simulink model "Dist_rej_lin"  (R2015b)
settings: Solver=VariableStepAuto  StartTime=0.0  StopTime=100  RelTol=1e-3
undefined symbols (not defined in the file): A, D
libraries: simulink x1
settings Model: Creator=Pramod  LastModifiedBy=Pramod

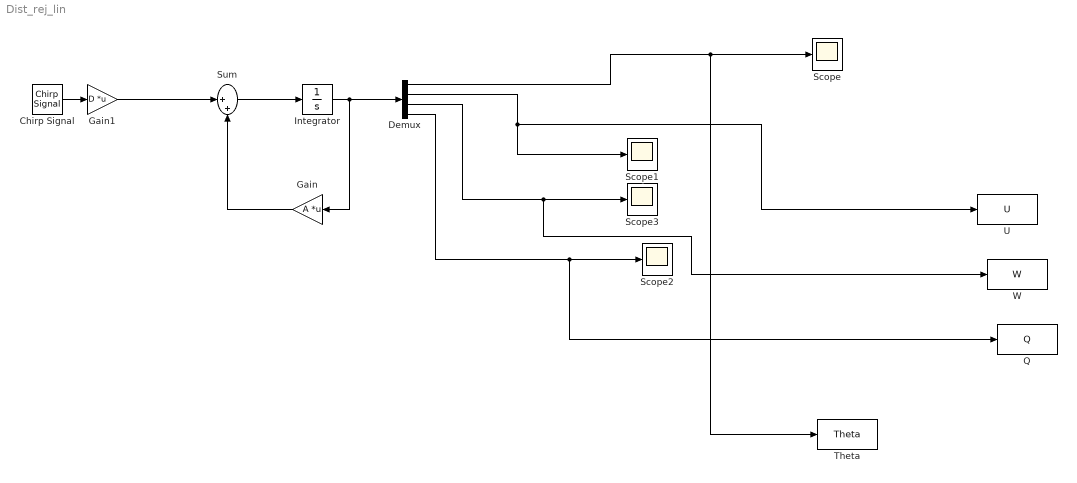
== system Dist_rej_lin ==
  Chirp Signal : simulink/Sources/Chirp Signal  f1=0.1  T=100  f2=1
  Demux : Demux
  Gain : Gain  Gain=A  Multiplication=Matrix(K*u)
  Gain1 : Gain  Gain=D  Multiplication=Matrix(K*u)
  Integrator : Integrator  InitialCondition="[39.5514    0.0872   -0.0000    1.3099]"
  Q : ToWorkspace  VariableName=Q  SaveFormat=Timeseries  SampleTime=-1
  Scope{,1..3} (4 alike) : Scope
  Sum : Sum  Inputs=|++
  Theta : ToWorkspace  VariableName=Theta  SaveFormat=Timeseries  SampleTime=-1
  U : ToWorkspace  VariableName=U  SaveFormat=Timeseries  SampleTime=-1
  W : ToWorkspace  VariableName=W  SaveFormat=Timeseries  SampleTime=-1
  wires:
  Integrator/1 -> Demux/1, Gain/1
  Sum/1 -> Integrator/1
  Gain/1 -> Sum/2
  Gain1/1 -> Sum/1
  Chirp Signal/1 -> Gain1/1
  Demux/1 -> Theta/1, Scope/1
  Demux/2 -> Scope1/1, U/1
  Demux/3 -> W/1, Scope3/1
  Demux/4 -> Q/1, Scope2/1
